simulink model "Fig257"  (R2014b)
settings: Solver=ode3  StartTime=0.0  StopTime=5.24288  FixedStep=2e-5  RelTol=1e-5
undefined symbols (not defined in the file): gcbh, rcfiltgaincompat
libraries: commfilt2 x2, commchan3 x1, commrandsrc2 x1
settings Model: Creator=Dennis Silage  LastModifiedBy=Silage
settings DataIOCC: SignalLoggingSaveFormat=ModelDataLogs
settings OptimizationCC: ExpressionDepthLimit=2147483647  InitFltsAndDblsToZero=on
settings DebuggingCC: UnderspecifiedInitializationDetection=Classic  MergeDetectMultiDrivingBlocksExec=none  SolverPrmCheckMsg=none  FcnCallInpInsideContextMsg=UseLocalSettings  StateNameClashWarn=warning
settings GRTTargetCC: CombineOutputUpdateFcns=off  GRTInterface=on

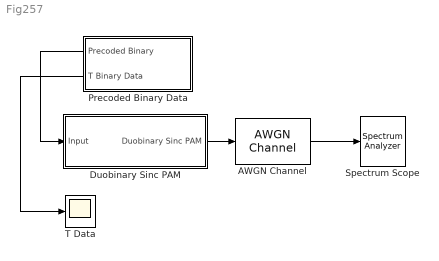
== system Fig257 ==
  AWGN Channel : commchan3/AWGN Channel  InputProcessing=Inherited (this choice will be removed - see release notes)  seed=randseed  noiseMode=Variance from mask  EbNodB=10  EsNodB=10  SNRdB=10  bitsPerSym=1  Ps=1  Tsym=1  variance=0
  Duobinary Sinc PAM : Subsystem
  Precoded Binary Data : Subsystem
  Spectrum Scope : SpectrumAnalyzer
  T Data : Scope
  wires:
  Precoded Binary Data/1(Precoded Binary) -> Duobinary Sinc PAM/1(Input)
  Duobinary Sinc PAM/1(Duobinary Sinc PAM) -> AWGN Channel/1
  Precoded Binary Data/2(T Binary Data) -> T Data/1
  AWGN Channel/1 -> Spectrum Scope/1

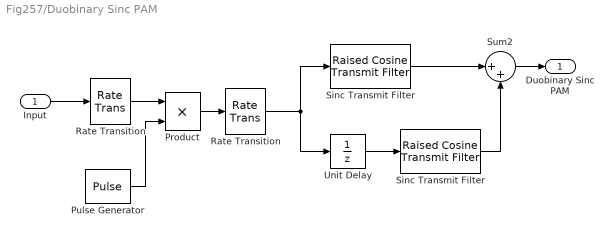
== system Fig257/Duobinary Sinc PAM ==
  Input : Inport
  " Rate Transition" : RateTransition  OutPortSampleTime=1e-3
  Product : Product  RndMeth=Zero
  Pulse Generator : DiscretePulseGenerator  PulseType=Time based  Period=1e-3  PulseWidth=2
  Rate Transition : RateTransition  OutPortSampleTime=2e-5
  Sinc Transmit Filter : commfilt2/Raised Cosine Transmit Filter  filtType=Normal  filtSpan=2*(4)  currentFiltSpan=2*(4)  D=4  R=0  sampMode=Mute  saveAsFlag=0  N=50  framing=Maintain input frame size  InputProcessing=Inherited (this choice will be removed - see release notes)  checkGain=User-specified  filterGain=(5)*rcfiltgaincompat(gcbh)  checkCoeff=off  variableName=rcTxFilt  launchFVT=off  roundingMode=Floor  overflowMode=off
  "Sinc Transmit Filter " : commfilt2/Raised Cosine Transmit Filter  filtType=Normal  filtSpan=2*(4)  currentFiltSpan=2*(4)  D=4  R=0  sampMode=Mute  saveAsFlag=0  N=50  framing=Maintain input frame size  InputProcessing=Inherited (this choice will be removed - see release notes)  checkGain=User-specified  filterGain=(5)*rcfiltgaincompat(gcbh)  checkCoeff=off  variableName=rcTxFilt1  launchFVT=off  roundingMode=Floor  overflowMode=off
  Sum2 : Sum  Inputs=|++
  Unit Delay : UnitDelay  SampleTime=-1
  Duobinary Sinc PAM : Outport
  wires:
  Rate Transition/1 -> Product/1
  Pulse Generator/1 -> Product/2
  " Rate Transition"/1 -> Sinc Transmit Filter/1, Unit Delay/1
  Product/1 -> " Rate Transition"/1
  Sum2/1 -> Duobinary Sinc PAM/1
  "Sinc Transmit Filter "/1 -> Sum2/2
  Sinc Transmit Filter/1 -> Sum2/1
  Unit Delay/1 -> "Sinc Transmit Filter "/1
  Input/1 -> Rate Transition/1

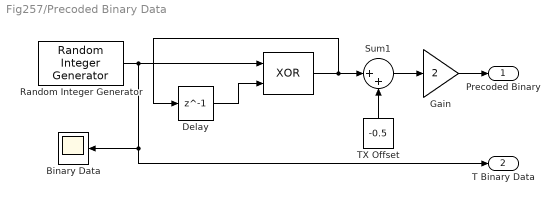
== system Fig257/Precoded Binary Data ==
  "  " : Logic  Operator=XOR  AllPortsSameDT=off  OutDataTypeStr=boolean
  Binary Data : Scope
      settings: TimeRange=0.05  YMin=-2  YMax=2  SaveName=ScopeData3
  "Delay " : Delay  DelayLength=1  InputProcessing=Inherited
  Gain : Gain  Gain=2
  Random Integer Generator : commrandsrc2/Random Integer Generator  mul=2  seed=randseed  Ts=1e-3  frameBased=off  sampPerFrame=50  orient=off  outDataType=boolean
  Sum1 : Sum  Inputs=|++
  TX Offset : Constant  Value=-0.5
  Precoded Binary : Outport
  T Binary Data : Outport  Port=2
  wires:
  Sum1/1 -> Gain/1
  TX Offset/1 -> Sum1/2
  Random Integer Generator/1 -> T Binary Data/1, Binary Data/1, "  "/1
  Gain/1 -> Precoded Binary/1
  "  "/1 -> Sum1/1, "Delay "/1
  "Delay "/1 -> "  "/2
